simulink model "Chp06Code01"  (R2019a)
settings: Solver=VariableStepAuto  StartTime=0.0  StopTime=10.0  RelTol=1e-3
settings Model: Creator=zhug  LastModifiedBy=ME456

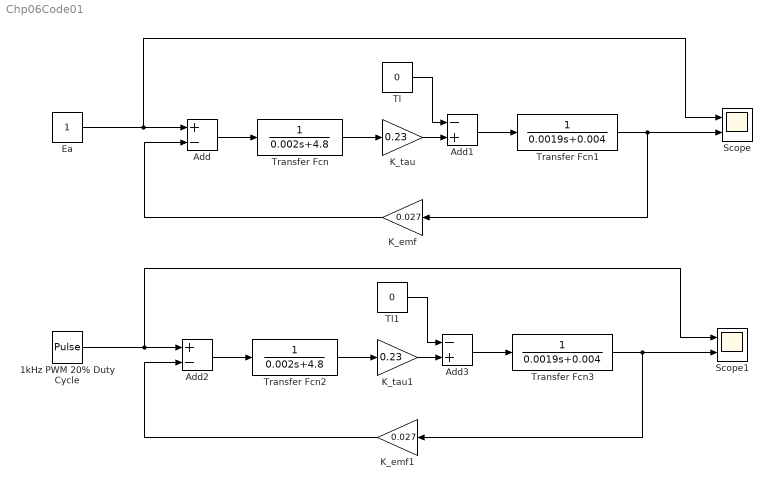
== system Chp06Code01 ==
  1kHz PWM 20% Duty Cycle : DiscretePulseGenerator  PulseType=Time based  Amplitude=5  Period=0.001  PulseWidth=20
  Add : Sum  Inputs=+-
  Add1 : Sum  Inputs=-+
  Add2 : Sum  Inputs=+-
  Add3 : Sum  Inputs=-+
  Ea : Constant
  K_emf : Gain  Gain=0.027
  K_emf1 : Gain  Gain=0.027
  K_tau : Gain  Gain=0.23
  K_tau1 : Gain  Gain=0.23
  Scope : Scope  NumInputPorts=2
  Scope1 : Scope  NumInputPorts=2
  Tl : Constant  Value=0
  Tl1 : Constant  Value=0
  Transfer Fcn : TransferFcn  Denominator=[0.002 4.8]
  Transfer Fcn1 : TransferFcn  Denominator=[0.0019 0.004]
  Transfer Fcn2 : TransferFcn  Denominator=[0.002 4.8]
  Transfer Fcn3 : TransferFcn  Denominator=[0.0019 0.004]
  wires:
  Ea/1 -> Scope/1, Add/1
  Add/1 -> Transfer Fcn/1
  Transfer Fcn/1 -> K_tau/1
  K_tau/1 -> Add1/2
  Tl/1 -> Add1/1
  Add1/1 -> Transfer Fcn1/1
  Transfer Fcn1/1 -> K_emf/1, Scope/2
  K_emf/1 -> Add/2
  1kHz PWM 20% Duty Cycle/1 -> Scope1/1, Add2/1
  Transfer Fcn3/1 -> K_emf1/1, Scope1/2
  Tl1/1 -> Add3/1
  Add3/1 -> Transfer Fcn3/1
  Transfer Fcn2/1 -> K_tau1/1
  Add2/1 -> Transfer Fcn2/1
  K_tau1/1 -> Add3/2
  K_emf1/1 -> Add2/2
